simulink model "SwingUp_2019"  (R2019b)
settings: Solver=ode1  StartTime=0.0  StopTime=inf  FixedStep=0.002  RelTol=1e-3  EnableMultiTasking=on
PostLoadFcn:
  | qc_set_target_type(getConfigSet(bdroot, 'QUARC Default Target Configuration'));
values from neighbouring files (symbols this model uses):
  g = th(8,1)    [NL_eqns_Disturbance.m]    (also in NL_eqns_EKF.m; StateFcn.m; computeFJacobian.m)
  J_a = th(3,1)    [NL_eqns_Disturbance.m]    (also in NL_eqns_EKF.m; StateFcn.m; computeFJacobian.m)
  K_g = th(9,1)    [NL_eqns_Disturbance.m]    (also in NL_eqns_EKF.m; StateFcn.m; computeFJacobian.m)
  k_m = th(13,1)    [NL_eqns_Disturbance.m]    (also in NL_eqns_EKF.m; StateFcn.m; computeFJacobian.m)
  l_p = th(5,1)    [NL_eqns_Disturbance.m]    (also in NL_eqns_EKF.m; StateFcn.m; computeFJacobian.m)
  m_p = th(6,1)    [NL_eqns_Disturbance.m]    (also in NL_eqns_EKF.m; StateFcn.m; computeFJacobian.m)
  r = th(7,1)    [NL_eqns_Disturbance.m]    (also in NL_eqns_EKF.m; StateFcn.m; computeFJacobian.m)
  Ts = 0.002    [StateFcn.m]
undefined symbols (not defined in the file or in its folder): A_ob, B_ob, c1_tau, C_ob, D_ob, E, HIL, id_param, Jp_prime, Ken_eta, Kpp, P0, qc_get_step_size, R, voltage_max, x0_KF, x0_ob
libraries: quarc_library x4
settings Model: SimulationMode=external  ExtModeTrigDuration=5000  Creator=CFulford  LastModifiedBy=utente
settings SolverCC: PositivePriorityOrder=on
settings DataIOCC: LimitDataPoints=on  SaveFormat=Array  SignalLoggingSaveFormat=ModelDataLogs  ReturnWorkspaceOutputs=off
settings OptimizationCC: ExpressionDepthLimit=2147483647  InitFltsAndDblsToZero=on  LifeSpan=inf
settings DebuggingCC: SaveWithParameterizedLinksMsg=none  UnderspecifiedInitializationDetection=Classic  MergeDetectMultiDrivingBlocksExec=none  SolverPrmCheckMsg=warning  MultiTaskDSMMsg=warning  MultiTaskCondExecSysMsg=none  FcnCallInpInsideContextMsg=warning  StateNameClashWarn=warning  SFUnexpectedBacktrackingDiag=warning  SFNoUnconditionalDefaultTransitionDiag=warning  SFExecutionAtInitializationDiag=none  ArithmeticOperatorsInVariantConditions=warning
settings HardwareCC: ProdBitPerPointer=32  ProdBitPerSizeT=32  ProdBitPerPtrDiffT=32  ProdLargestAtomicFloat=None  ProdIntDivRoundTo=Undefined  ProdEndianess=Unspecified  ProdWordSize=32  ProdHWDeviceType=32-bit Generic
settings ModelReferenceCC: PropagateSignalLabelsOutOfModel=off
settings SFSimCC: SimUseLocalCustomCode=off  CustomCodeUndefinedFunction=UseInterfaceOnly
settings RTWCC: Description=QUARC Win64 Target  SystemTargetFile=quarc_win64.tlc  TemplateMakefile=quarc_default_tmf  RTWUseLocalCustomCode=off
settings CodeAppCC: StateflowObjectComments=on
settings STFCustomTargetCC: TargetPreCompLibLocation=C:\PROGRA~3\QUARC\lib\2019b\win64\release  ConcurrentExecutionCompliant=on  CombineOutputUpdateFcns=on  CPPClassGenCompliant=on  SystemTargetFile=quarc_win64.tlc
settings GRTTargetCC: TargetPreCompLibLocation=C:\PROGRA~3\QUARC\lib\2019b\win64\release  TargetLangStandard=C89/C90 (ANSI)  ParMdlRefBuildCompliant=off  CompOptLevelCompliant=off  MatFileLogging=off  UseToolchainInfoCompliant=off  ExtMode=on  ExtModeMexFile=quarc_comm
settings ConfigComp: CovMetricSettings=dw  CovSaveCumulativeToWorkspaceVar=on  CovSaveSingleToWorkspaceVar=on  CovExternalEMLEnable=off  CovSFcnEnable=off

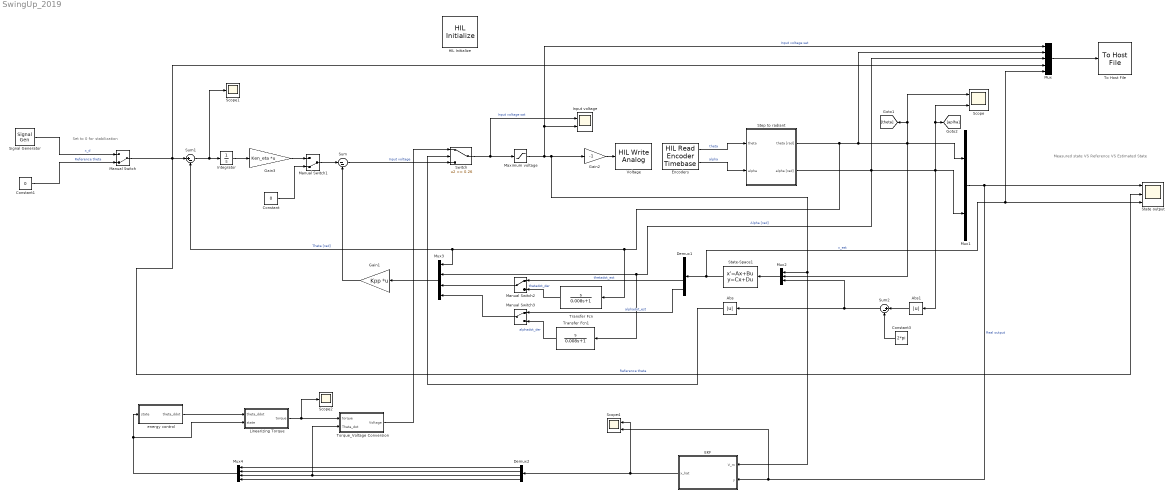
== system SwingUp_2019 ==
  note: Set to 0 for stabilization
  note: Measured state VS Reference VS Estimated State
  Abs : Abs
  Abs1 : Abs
  Constant : Constant  Value=0
  Constant1 : Constant  Value=0
  Constant3 : Constant  Value=2*pi
  Demux1 : Demux
  Demux2 : Demux
  EKF : Subsystem
  Encoders : quarc_library/Data Acquisition/Generic/Timebases/HIL Read Encoder Timebase  object_name=HIL-1  clock=0  channels=[0:1]  samples_in_buffer=max(ceil(1/qc_get_step_size), 1)  active=on  vector_output=off  data_type_mode=Inherit via back propagation  data_type=double
  Gain1 : Gain  Gain=Kpp  Multiplication=Matrix(K*u) (u vector)
  Gain2 : Gain  Gain=-1
  Gain3 : Gain  Gain=Ken_eta  Multiplication=Matrix(K*u) (u vector)
  HIL Initialize : quarc_library/Data Acquisition/Generic/Configuration/HIL Initialize  Priority=-99  object_name=HIL-1  board_type=q2_usb  board_number=0  board_options=d0=digital;d1=digital;led=auto;update_rate=normal;decimation=1  exclusive=off  active=off  hardware_clocks=[0]  clock_modes=[]  initial_clock_frequencies=[]  set_clock_params_at_start=off  set_clock_params_at_switch_in=off  set_clock_frequencies_at_start=off  set_clock_frequencies_at_switch_in=off  analog_input_channels=[0:1]  analog_input_configurations=[]  analog_input_maximums=10  analog_input_minimums=-10  set_analog_input_params_at_start=on  set_analog_input_params_at_switch_in=off  analog_output_channels=[0:1]  analog_output_maximums=10  analog_output_minimums=-10  initial_analog_outputs=[0]  final_analog_outputs=[0]  watchdog_analog_outputs=0  set_analog_output_params_at_start=on  set_analog_output_params_at_switch_in=off  set_analog_outputs_at_start=on  set_analog_outputs_at_switch_in=off  set_analog_outputs_at_terminate=on  set_analog_outputs_at_switch_out=off  set_analog_outputs_on_watchdog=off  digital_input_channels=[]  digital_output_channels=[]  digital_output_configuration=[]  initial_digital_outputs=[1]  final_digital_outputs=[1]  watchdog_digital_outputs=[1]  set_digital_output_params_at_start=off  set_digital_output_params_at_switch_in=off  set_digital_outputs_at_start=on  set_digital_outputs_at_switch_in=off  set_digital_outputs_at_terminate=on  set_digital_outputs_at_switch_out=off  set_digital_outputs_on_watchdog=off  encoder_channels=[0:1]  quadrature=[4]  encoder_filter_frequency=[]  initial_encoder_counts=[0]  set_encoder_params_at_start=on  set_encoder_params_at_switch_in=off  set_encoder_counts_at_start=on  set_encoder_counts_at_switch_in=off  pwm_channels=[]  pwm_modes=[0]  pwm_frequency=1/0.020  pwm_configuration=[]  pwm_alignment=[]  pwm_polarity=[]  pwm_leading_deadband=[]  pwm_trailing_deadband=[]  initial_pwm_outputs=[0]  final_pwm_outputs=[0]  watchdog_pwm_outputs=[0]  set_pwm_params_at_start=on  set_pwm_params_at_switch_in=off  set_pwm_outputs_at_start=on  set_pwm_outputs_at_switch_in=off  set_pwm_outputs_at_terminate=on  set_pwm_outputs_at_switch_out=off  set_pwm_outputs_on_watchdog=off  other_output_channels=[]  initial_other_outputs=[]  final_other_outputs=[]  watchdog_other_outputs=[]  set_other_outputs_at_start=off  set_other_outputs_at_switch_in=off  set_other_outputs_at_terminate=off  set_other_outputs_at_switch_out=off  set_other_outputs_on_watchdog=off
  Input voltage : Scope  NumInputPorts=2
  Integrator : Integrator  LimitOutput=on  UpperSaturationLimit=3  LowerSaturationLimit=-3
  Linearizing Torque : Subsystem
  Manual Switch : ManualSwitch  CurrentSetting=0
  Manual Switch1 : ManualSwitch  CurrentSetting=0
  Manual Switch2 : ManualSwitch
  Manual Switch3 : ManualSwitch
  Maximum voltage : Saturate  UpperLimit=voltage_max  LowerLimit=-voltage_max
  Mux : Mux  Inputs=5
  Mux1 : Mux  Inputs=2
  Mux2 : Mux  Inputs=3
  Mux3 : Mux
  Mux4 : Mux
  Scope : Scope  NumInputPorts=2
  Scope1 : Scope
  Scope2 : Scope
  Scope4 : Scope  NumInputPorts=2
  Signal Generator : SignalGenerator  WaveForm=square  Amplitude=0.3  Frequency=0.1
  State output : Scope  NumInputPorts=3
  State-Space1 : StateSpace  A=A_ob  B=B_ob  C=C_ob  D=D_ob  InitialCondition=x0_ob
  Step to radiant : Subsystem
  Sum : Sum  Inputs=|--
  Sum1 : Sum  Inputs=|+-
  Sum2 : Sum  Inputs=|+-
  Switch : Switch  Threshold=0.26
  To Host File : quarc_library/Sinks/To Host/To Host File  file_name=data_%{date}_%{time}.mat  variable_name=data_%{date}_%{time}  decimation=1  sample_time=-1  file_format=MAT-file v.5  options=No header or footer  append=off  final_file_name=data_18-Apr-2023_18-40-39.mat  bitrate=2000000
  Torque_Voltage Conversion : Subsystem
  Transfer Fcn : TransferFcn  Numerator=[1 0]  Denominator=[0.008 1]
  Transfer Fcn1 : TransferFcn  Numerator=[1 0]  Denominator=[0.008 1]
  Voltage : quarc_library/Data Acquisition/Generic/Immediate I//O/HIL Write Analog  object_name=HIL-1  channels=0  sample_time=-1  active=off  vector_input=off
  energy control : Subsystem
  wires:
  Mux/1 -> To Host File/1
  Sum/1 -> Switch/3  "Input voltage"
  Gain2/1 -> Voltage/1
  Encoders/1 -> Step to radiant/1(theta)  "theta"
  Encoders/2 -> Step to radiant/2(alpha)  "alpha"
  Signal Generator/1 -> Manual Switch/1  "x_d"
  Step to radiant/1(theta [rad]) -> Transfer Fcn/1, Sum1/2, Mux3/1, Mux/2, Mux2/2, Mux1/1, Scope/1, [theta]  "Theta [rad]"
  Step to radiant/2(alpha [rad]) -> Mux3/2, Transfer Fcn1/1, Mux/3, Abs1/1, Scope/2, [aplha], Mux1/2  "Alpha [rad]"
  Mux1/1 -> Scope4/2, EKF/2(y), State output/1  "Real output"
  Manual Switch/1 -> Mux/4, State output/2, Sum1/1  "Reference theta"
  Maximum voltage/1 -> Mux/1, Input voltage/2, EKF/1(V_m), Mux2/1, Gain2/1  "Input voltage sat"
  Mux2/1 -> State-Space1/1
  Mux3/1 -> Gain1/1
  State-Space1/1 -> Demux1/1, Mux/5, State output/3  "x_est"
  Integrator/1 -> Gain3/1
  Gain1/1 -> Sum/2
  Sum1/1 -> Scope1/1, Integrator/1
  Gain3/1 -> Manual Switch1/1
  Constant/1 -> Manual Switch1/2
  Manual Switch1/1 -> Sum/1
  Demux1/3 -> Manual Switch2/1  "thetadot_est"
  Demux1/4 -> Manual Switch3/1  "alphadot_est"
  Transfer Fcn/1 -> Manual Switch2/2  "thetadot_der"
  Transfer Fcn1/1 -> Manual Switch3/2  "alphadot_der"
  Manual Switch2/1 -> Mux3/3
  Manual Switch3/1 -> Mux3/4
  Constant1/1 -> Manual Switch/2  "Reference theta"
  Mux4/1 -> energy control/1(state), Linearizing Torque/2(state)
  Demux2/2 -> Mux4/2
  Demux2/4 -> Mux4/4
  Linearizing Torque/1(torque) -> Torque_Voltage Conversion/1(torque), Scope2/1
  energy control/1(theta_ddot) -> Linearizing Torque/1(theta_ddot)
  EKF/1(x_hat) -> Demux2/1, Scope4/1
  Demux2/1 -> Mux4/1
  Demux2/3 -> Mux4/3, Torque_Voltage Conversion/2(Theta_dot)
  Switch/1 -> Maximum voltage/1, Input voltage/1  "Input voltage sat"
  Torque_Voltage Conversion/1(Voltage) -> Switch/1
  Abs1/1 -> Sum2/1
  Constant3/1 -> Sum2/2
  Sum2/1 -> Mux2/3, Abs/1
  Abs/1 -> Switch/2

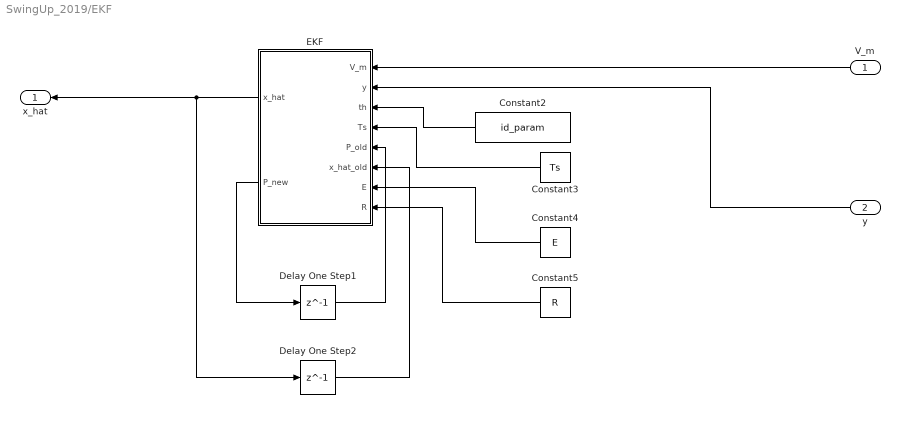
== system SwingUp_2019/EKF ==
  V_m : Inport
  y : Inport  Port=2
  Constant2 : Constant  Value=id_param
  Constant3 : Constant  Value=Ts
  Constant4 : Constant  Value=E
  Constant5 : Constant  Value=R
  Delay One Step1 : Delay  DelayLength=1  InitialCondition=P0  SampleTime=Ts
  Delay One Step2 : Delay  DelayLength=1  InitialCondition=x0_KF  SampleTime=Ts
  EKF : MATLAB Function  TreatAsAtomicUnit=on
  x_hat : Outport
  wires:
  Constant5/1 -> EKF/8(R)
  y/1 -> EKF/2(y)
  Delay One Step2/1 -> EKF/6(x_hat_old)
  Constant2/1 -> EKF/3(th)
  EKF/1(x_hat) -> Delay One Step2/1, x_hat/1
  V_m/1 -> EKF/1(V_m)
  Constant3/1 -> EKF/4(Ts)
  Constant4/1 -> EKF/7(E)
  Delay One Step1/1 -> EKF/5(P_old)
  EKF/2(P_new) -> Delay One Step1/1

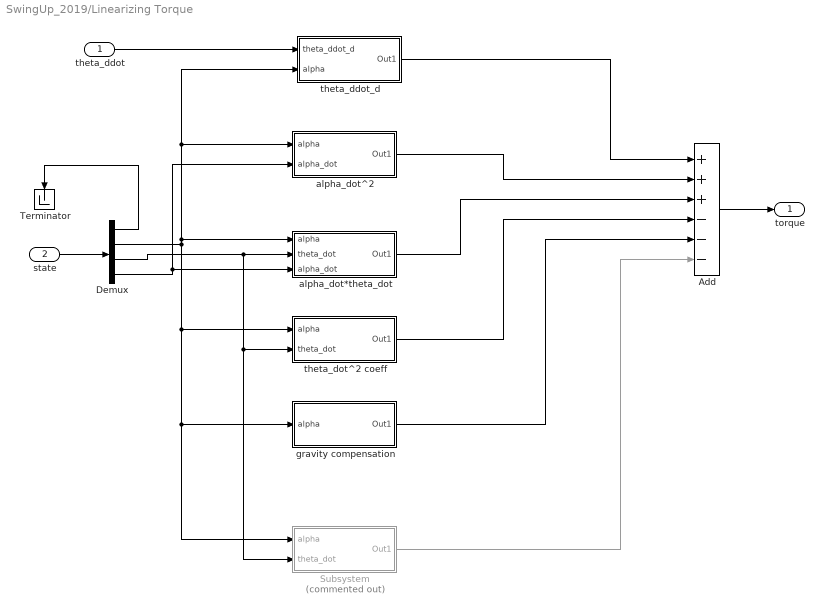
== system SwingUp_2019/Linearizing Torque ==
  theta_ddot : Inport
  state : Inport  Port=2
  Add : Sum  Inputs=+++---
  Demux : Demux
  Subsystem : Subsystem  Commented=on
  Terminator : Terminator
  alpha_dot*theta_dot : Subsystem
  alpha_dot^2 : Subsystem
  gravity compensation : Subsystem
  theta_ddot_d : Subsystem
  theta_dot^2 coeff : Subsystem
  torque : Outport
  wires:
  Add/1 -> torque/1
  gravity compensation/1(Out1) -> Add/5
  theta_dot^2 coeff/1(Out1) -> Add/4
  alpha_dot*theta_dot/1(Out1) -> Add/3
  alpha_dot^2/1(Out1) -> Add/2
  theta_ddot_d/1(Out1) -> Add/1
  theta_ddot/1 -> theta_ddot_d/1(theta_ddot_d)
  state/1 -> Demux/1
  Demux/1 -> Terminator/1
  Demux/2 -> Subsystem/1(alpha), gravity compensation/1(alpha), theta_dot^2 coeff/1(alpha), alpha_dot*theta_dot/1(alpha), alpha_dot^2/1(alpha), theta_ddot_d/2(alpha)
  Demux/3 -> theta_dot^2 coeff/2(theta_dot), Subsystem/2(theta_dot), alpha_dot*theta_dot/2(theta_dot)
  Demux/4 -> alpha_dot*theta_dot/3(alpha_dot), alpha_dot^2/2(alpha_dot)
  Subsystem/1(Out1) -> Add/6

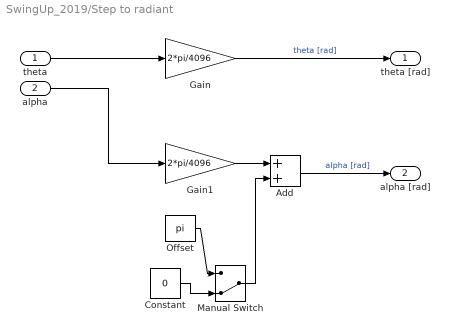
== system SwingUp_2019/Step to radiant ==
  theta : Inport
  alpha : Inport  Port=2
  Add : Sum
  Constant : Constant  Value=0
  Gain : Gain  Gain=2*pi/4096
  Gain1 : Gain  Gain=2*pi/4096
  Manual Switch : ManualSwitch  CurrentSetting=0
  Offset : Constant  Value=pi
  theta [rad] : Outport
  alpha [rad] : Outport  Port=2
  wires:
  Gain1/1 -> Add/1
  Gain/1 -> theta [rad]/1  "theta [rad]"
  Add/1 -> alpha [rad]/1  "alpha [rad]"
  theta/1 -> Gain/1
  alpha/1 -> Gain1/1
  Offset/1 -> Manual Switch/1
  Constant/1 -> Manual Switch/2
  Manual Switch/1 -> Add/2

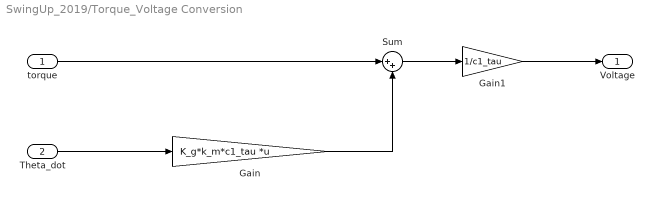
== system SwingUp_2019/Torque_Voltage Conversion ==
  torque : Inport
  Theta_dot : Inport  Port=2
  Gain : Gain  Gain=K_g*k_m*c1_tau  Multiplication=Matrix(K*u)
  Gain1 : Gain  Gain=1/c1_tau
  Sum : Sum  Inputs=|++
  Voltage : Outport
  wires:
  Theta_dot/1 -> Gain/1
  Gain1/1 -> Voltage/1
  Sum/1 -> Gain1/1
  Gain/1 -> Sum/2
  torque/1 -> Sum/1

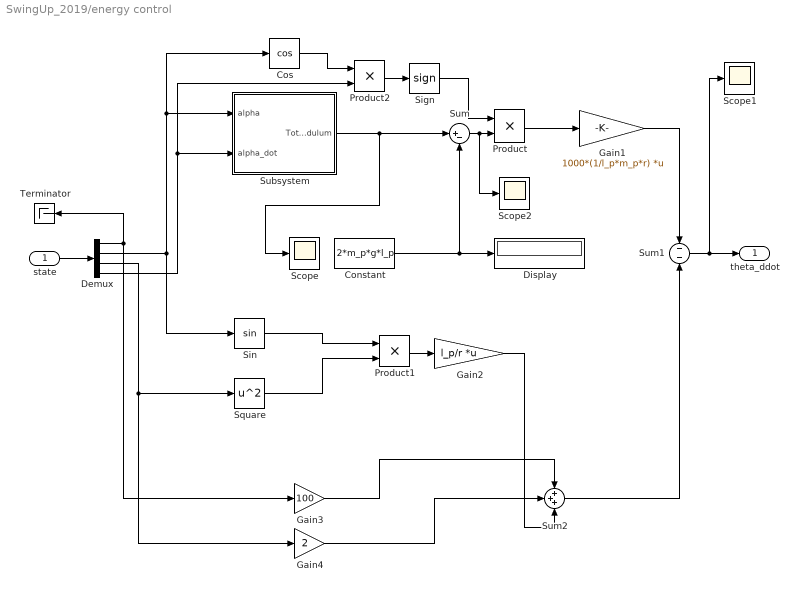
== system SwingUp_2019/energy control ==
  state : Inport
  Constant : Constant  Value=2*m_p*g*l_p
  Cos : Trigonometry  Operator=cos
  Demux : Demux
  Display : Display
  Gain1 : Gain  Gain=1000*(1/l_p*m_p*r)  Multiplication=Matrix(K*u)
  Gain2 : Gain  Gain=l_p/r  Multiplication=Matrix(K*u)
  Gain3 : Gain  Gain=100
  Gain4 : Gain  Gain=2
  Product : Product
  Product1 : Product
  Product2 : Product
  Scope : Scope
  Scope1 : Scope
  Scope2 : Scope
  Sign : Signum
  Sin : Trigonometry
  Square : Math  Operator=square  SignedPower=off  SaturateOnIntegerOverflow=on
  Subsystem : Subsystem
  Sum : Sum  Inputs=|+-
  Sum1 : Sum  Inputs=--
  Sum2 : Sum  Inputs=+++
  Terminator : Terminator
  theta_ddot : Outport
  wires:
  state/1 -> Demux/1
  Demux/2 -> Sin/1, Subsystem/1(alpha), Cos/1
  Demux/4 -> Subsystem/2(alpha_dot), Product2/2
  Cos/1 -> Product2/1
  Product/1 -> Gain1/1
  Gain2/1 -> Sum2/3
  Product1/1 -> Gain2/1
  Demux/3 -> Square/1, Gain4/1
  Demux/1 -> Gain3/1, Terminator/1
  Sin/1 -> Product1/1
  Square/1 -> Product1/2
  Product2/1 -> Sign/1
  Subsystem/1(Total Energy Pendulum) -> Sum/1, Scope/1
  Sum1/1 -> Scope1/1, theta_ddot/1
  Gain3/1 -> Sum2/1
  Gain4/1 -> Sum2/2
  Sum2/1 -> Sum1/2
  Gain1/1 -> Sum1/1
  Sum/1 -> Scope2/1, Product/2
  Constant/1 -> Display/1, Sum/2
  Sign/1 -> Product/1

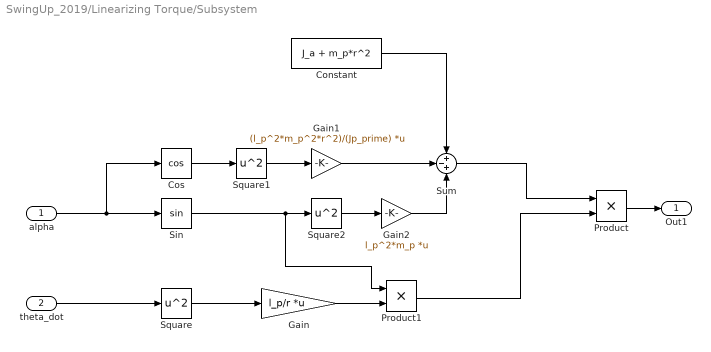
== system SwingUp_2019/Linearizing Torque/Subsystem ==
  alpha : Inport
  theta_dot : Inport  Port=2
  Constant : Constant  Value=J_a + m_p*r^2
  Cos : Trigonometry  Operator=cos
  Gain : Gain  Gain=l_p/r  Multiplication=Matrix(K*u)
  Gain1 : Gain  Gain=(l_p^2*m_p^2*r^2)/(Jp_prime)  Multiplication=Matrix(K*u)
  Gain2 : Gain  Gain=l_p^2*m_p  Multiplication=Matrix(K*u)
  Product : Product
  Product1 : Product
  Sin : Trigonometry
  Square : Math  Operator=square  SignedPower=off  SaturateOnIntegerOverflow=on
  Square1 : Math  Operator=square  SignedPower=off  SaturateOnIntegerOverflow=on
  Square2 : Math  Operator=square  SignedPower=off  SaturateOnIntegerOverflow=on
  Sum : Sum  Inputs=+-+
  Out1 : Outport
  wires:
  theta_dot/1 -> Square/1
  alpha/1 -> Sin/1, Cos/1
  Square/1 -> Gain/1
  Product/1 -> Out1/1
  Gain/1 -> Product1/2
  Sin/1 -> Square2/1, Product1/1
  Cos/1 -> Square1/1
  Square1/1 -> Gain1/1
  Gain1/1 -> Sum/2
  Square2/1 -> Gain2/1
  Gain2/1 -> Sum/3
  Constant/1 -> Sum/1
  Sum/1 -> Product/1
  Product1/1 -> Product/2

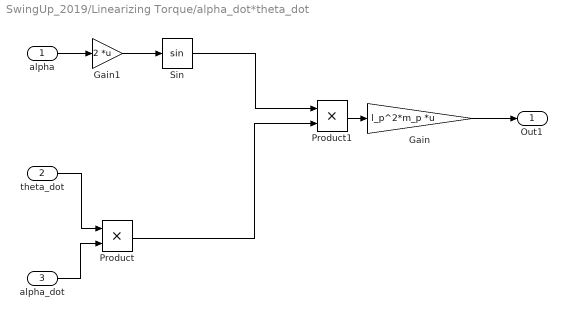
== system SwingUp_2019/Linearizing Torque/alpha_dot*theta_dot ==
  alpha : Inport
  theta_dot : Inport  Port=2
  alpha_dot : Inport  Port=3
  Gain : Gain  Gain=l_p^2*m_p  Multiplication=Matrix(K*u)
  Gain1 : Gain  Gain=2  Multiplication=Matrix(K*u)
  Product : Product
  Product1 : Product
  Sin : Trigonometry
  Out1 : Outport
  wires:
  theta_dot/1 -> Product/1
  alpha_dot/1 -> Product/2
  Gain/1 -> Out1/1
  Product1/1 -> Gain/1
  Product/1 -> Product1/2
  alpha/1 -> Gain1/1
  Gain1/1 -> Sin/1
  Sin/1 -> Product1/1

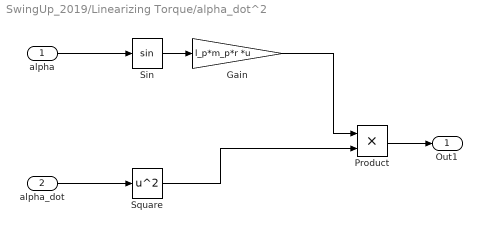
== system SwingUp_2019/Linearizing Torque/alpha_dot^2 ==
  alpha : Inport
  alpha_dot : Inport  Port=2
  Gain : Gain  Gain=l_p*m_p*r  Multiplication=Matrix(K*u)
  Product : Product
  Sin : Trigonometry
  Square : Math  Operator=square  SignedPower=off  SaturateOnIntegerOverflow=on
  Out1 : Outport
  wires:
  alpha_dot/1 -> Square/1
  Product/1 -> Out1/1
  Square/1 -> Product/2
  alpha/1 -> Sin/1
  Sin/1 -> Gain/1
  Gain/1 -> Product/1

== system SwingUp_2019/Linearizing Torque/gravity compensation ==
  alpha : Inport
  Cos : Trigonometry  Operator=cos
  Gain : Gain  Gain=(g*l_p^2*m_p^2*r)/Jp_prime  Multiplication=Matrix(K*u)
  Product : Product
  Sin : Trigonometry
  Out1 : Outport
  wires:
  Gain/1 -> Out1/1
  Product/1 -> Gain/1
  Cos/1 -> Product/1
  Sin/1 -> Product/2
  alpha/1 -> Cos/1, Sin/1

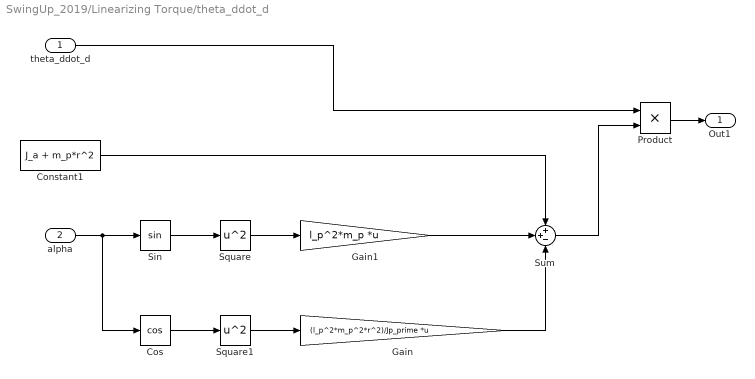
== system SwingUp_2019/Linearizing Torque/theta_ddot_d ==
  theta_ddot_d : Inport
  alpha : Inport  Port=2
  Constant1 : Constant  Value=J_a + m_p*r^2
  Cos : Trigonometry  Operator=cos
  Gain : Gain  Gain=(l_p^2*m_p^2*r^2)/Jp_prime  Multiplication=Matrix(K*u)
  Gain1 : Gain  Gain=l_p^2*m_p  Multiplication=Matrix(K*u)
  Product : Product
  Sin : Trigonometry
  Square : Math  Operator=square  SignedPower=off  SaturateOnIntegerOverflow=on
  Square1 : Math  Operator=square  SignedPower=off  SaturateOnIntegerOverflow=on
  Sum : Sum  Inputs=++-
  Out1 : Outport
  wires:
  Product/1 -> Out1/1
  theta_ddot_d/1 -> Product/1
  Sin/1 -> Square/1
  alpha/1 -> Sin/1, Cos/1
  Cos/1 -> Square1/1
  Square/1 -> Gain1/1
  Square1/1 -> Gain/1
  Constant1/1 -> Sum/1
  Gain1/1 -> Sum/2
  Gain/1 -> Sum/3
  Sum/1 -> Product/2

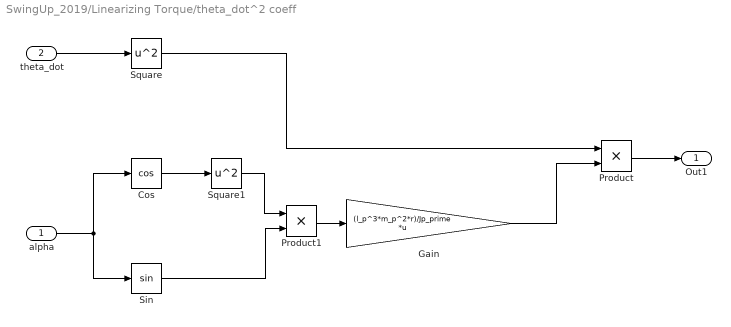
== system SwingUp_2019/Linearizing Torque/theta_dot^2 coeff ==
  alpha : Inport
  theta_dot : Inport  Port=2
  Cos : Trigonometry  Operator=cos
  Gain : Gain  Gain=(l_p^3*m_p^2*r)/Jp_prime  Multiplication=Matrix(K*u)
  Product : Product
  Product1 : Product
  Sin : Trigonometry
  Square : Math  Operator=square  SignedPower=off  SaturateOnIntegerOverflow=on
  Square1 : Math  Operator=square  SignedPower=off  SaturateOnIntegerOverflow=on
  Out1 : Outport
  wires:
  theta_dot/1 -> Square/1
  Product/1 -> Out1/1
  Square/1 -> Product/1
  Cos/1 -> Square1/1
  alpha/1 -> Sin/1, Cos/1
  Product1/1 -> Gain/1
  Square1/1 -> Product1/1
  Sin/1 -> Product1/2
  Gain/1 -> Product/2

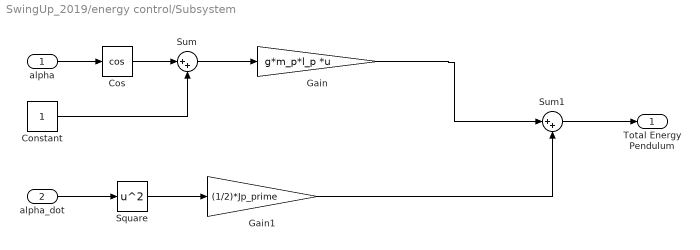
== system SwingUp_2019/energy control/Subsystem ==
  alpha : Inport
  alpha_dot : Inport  Port=2
  Constant : Constant
  Cos : Trigonometry  Operator=cos
  Gain : Gain  Gain=g*m_p*l_p  Multiplication=Matrix(K*u)
  Gain1 : Gain  Gain=(1/2)*Jp_prime
  Square : Math  Operator=square  SignedPower=off  SaturateOnIntegerOverflow=on
  Sum : Sum  Inputs=|++
  Sum1 : Sum  Inputs=|++
  Total Energy Pendulum : Outport
  wires:
  alpha/1 -> Cos/1
  Cos/1 -> Sum/1
  Constant/1 -> Sum/2
  Sum/1 -> Gain/1
  Sum1/1 -> Total Energy Pendulum/1
  Gain/1 -> Sum1/1
  alpha_dot/1 -> Square/1
  Square/1 -> Gain1/1
  Gain1/1 -> Sum1/2

== matlab function SwingUp_2019/EKF/EKF ==
  data: V_m input; x_hat output; y input; th input; Ts input; P_old input; x_hat_old input; E input; R input; P_new output
function [x_hat,P_new] = fcn(V_m,y,th,Ts,P_old,x_hat_old,E,R)
% INPUTS
% V_m: input variable, the voltage
% y: measured state
% th: vector of dynamical parameters of the pendulum
% Ts: sampling time for the DT model used in the filter
% P_old: previous state covariance matrix
% x_hat_old: previous state 
% E process covariance matrix
% R measurement covariance matrix
param = th;
%{=============== PREDICTION =============}%
x = x_hat_old + Ts*NL_eqns_EKF(x_hat_old,V_m,param); % FW Euler simulation one step
F_k = computeFJacobian(Ts,x(1),x(2),x(3),x(4),V_m,param); % jacobian matrix
P_temp = F_k*P_old*(F_k') + E; % update covariance matrix
yK = [x(1);x(2)]; % compute output prediction estimate

%{========================================}%
%{=============== CORRECTION =============}%

H = eye(2,4); % output matrix
I = eye(4);
% innovation
e =  y - yK; % difference between real meas. and predicted output
Ht = H'; % H transposed, compute just once and use 2 times
S = H*P_temp*Ht + R;  % % residual covariance

% near optimal Kalman Gain
K =  (P_temp*Ht)/S;

% updated state estimate
x_hat = x + K*e; % feedback correction
% updated covariance estimate
P_new = (I-K*H)*P_temp;
